simulink model "hydraulic_nonlin_stud"  (R2025b)
settings: Solver=ode4  StartTime=0.0  StopTime=30  FixedStep=0.001  RelTol=1e-3
values from neighbouring files (symbols this model uses):
  A = real(A)    [untitled.m]
  B = real(B)    [untitled.m]
  C = [1 0 0 0]    [untitled.m]
  D = 0    [untitled.m]
  k = real(k)    [untitled.m]
  N = real(N)    [untitled.m]
libraries: simulink x1
settings Model: Creator=Zsofi  LastModifiedBy=User
settings SolverCC: AlgebraicLoopSolver=TrustRegion
settings DataIOCC: SaveFormat=StructureWithTime  ReturnWorkspaceOutputs=off
settings OptimizationCC: LifeSpan=inf
settings DebuggingCC: FcnCallInpInsideContextMsg=warning  UnconnectedInputMsg=warning  UnconnectedOutputMsg=warning  UnconnectedLineMsg=warning  SFExecutionAtInitializationDiag=none  ArithmeticOperatorsInVariantConditions=warning
settings HardwareCC: ProdBitPerSizeT=32.0  ProdBitPerPtrDiffT=32.0  ProdWordSize=32.0  ProdHWDeviceType=Specified
settings ModelReferenceCC: EnableRefExpFcnMdlSchedulingChecks=on
settings SFSimCC: SimUseLocalCustomCode=off  CustomCodeUndefinedFunction=UseInterfaceOnly
settings RTWCC: RTWUseLocalCustomCode=off  GPUComputeCapability=3.5
settings CodeAppCC: StateflowObjectComments=on

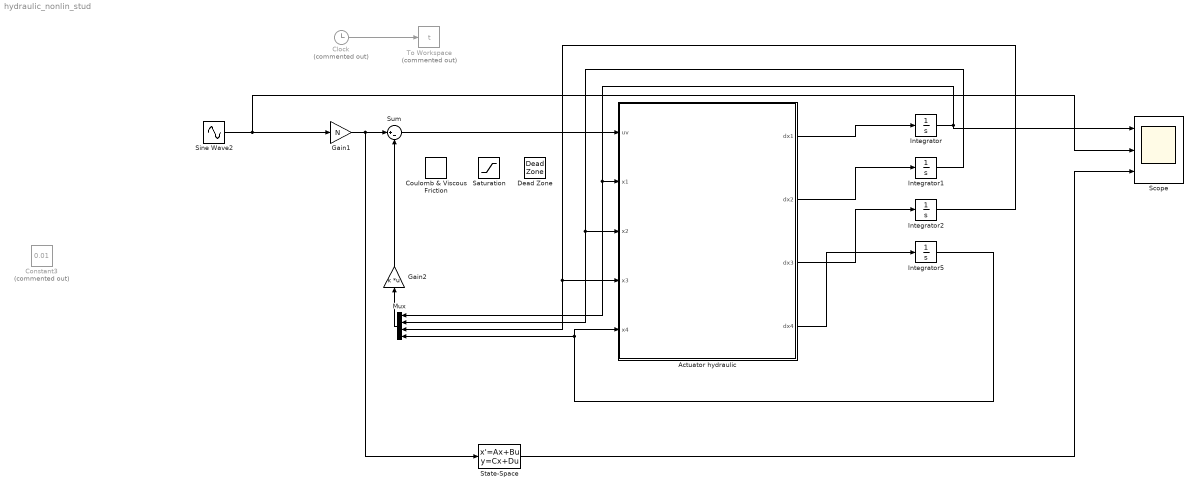
== system hydraulic_nonlin_stud ==
  Actuator hydraulic : MATLAB Function  TreatAsAtomicUnit=on
  Clock : Clock  Commented=on
  Constant3 : Constant  Commented=on  Value=0.01
  Coulomb & Viscous Friction : simulink/Discontinuities/Coulomb & Viscous Friction  offset=[0.005]  gain=1
  Dead Zone : DeadZone  LowerValue=-0.005  UpperValue=0.005
  Gain1 : Gain  Gain=N
  Gain2 : Gain  Gain=k  Multiplication=Matrix(K*u)
  Integrator{,1..2,5} (4 alike) : Integrator
  Mux : Mux
  Saturation : Saturate  UpperLimit=0.1  LowerLimit=-0.1
  Scope : Scope  NumInputPorts=3
      settings: ActiveDisplayYMinimum=-0.024999999679969208  ActiveDisplayYMaximum=0.024999999961916909
  Sine Wave2 : Sin  Amplitude=0.02  Frequency=10  SampleTime=0
  State-Space : StateSpace  A=A-B*k  B=B  C=C  D=D  InitialCondition=0
  Sum : Sum  Inputs=|+-
  To Workspace : ToWorkspace  Commented=on  VariableName=t  SampleTime=-1
  wires:
  Clock/1 -> To Workspace/1
  Actuator hydraulic/1(dx1) -> Integrator/1
  Integrator/1 -> Scope/1, Mux/1, Actuator hydraulic/2(x1)
  Integrator1/1 -> Mux/2, Actuator hydraulic/3(x2)
  Actuator hydraulic/2(dx2) -> Integrator1/1
  Integrator2/1 -> Actuator hydraulic/4(x3), Mux/3
  Actuator hydraulic/3(dx3) -> Integrator2/1
  Sine Wave2/1 -> Scope/2, Gain1/1
  Actuator hydraulic/4(dx4) -> Integrator5/1
  Integrator5/1 -> Mux/4, Actuator hydraulic/5(x4)
  Gain1/1 -> State-Space/1, Sum/1
  Mux/1 -> Gain2/1
  Gain2/1 -> Sum/2
  Sum/1 -> Actuator hydraulic/1(uv)
  State-Space/1 -> Scope/3

== matlab function hydraulic_nonlin_stud/Actuator hydraulic ==
  data: uv input; dx1 output; dx2 output; dx3 output; dx4 output; x1 input; x2 input; x3 input; x4 input
function [dx1, dx2, dx3, dx4] = fcn(uv, x1, x2, x3, x4)
M = 10.8;    
Bv = 13.1;   
L0 = 0.1635; 
b = 1.04;    
Kg = 1.035;  
gamma = 1.4; 
R = 287;     
T = 293;     
RT = R*T;
Patm = 101325; 
Ps = 600000;   
P0 = 300000;   
cv = 0.024;    

%iesiri
dx1 = 0; dx2 = 0; dx3 = 0; dx4 = 0;

% limite sigure pentru comanda de intrare directa
if uv > 10
    uv_safe = 10;     % limitare +10V
elseif uv < -10
    uv_safe = -10;    % limitare -10V
else
    uv_safe = uv;     % comanda in interval sigur
end

if x1 > 0.05
    x1_limited = 0.05;   % +5 cm
elseif x1 < -0.05
    x1_limited = -0.05;  % -5 cm
else
    x1_limited = x1;     
end

La = L0 + x1_limited; 
Lb = L0 - x1_limited;

Va = max(1e-4, (La * (b^2 - (La^2))) / Kg);
Vb = max(1e-4, (Lb * (b^2 - (Lb^2))) / Kg); 

dVadx = (b^2 - 3*(La^2)) / Kg;
dVbdx = -(b^2 - 3*(Lb^2)) / Kg; 

% debite si presiuni
% se imparte cu 1e5 pt a se potrivi cu unitatile
qmA = cv * uv_safe * sqrt(max(0, Ps - P0)/1e5);
qmB = -cv * uv_safe * sqrt(max(0, P0 - Patm)/1e5);

% dinamica presiunilor individuale
dPa = (gamma * RT * qmA) / Va - (gamma * P0 / Va) * dVadx * x2;
dPb = (gamma * RT * qmB) / Vb - (gamma * P0 / Vb) * dVbdx * x2; 
dPd = dPa - dPb;

% dinamica mecanica
F_pneuma = x4 * dVadx;
dacc_mecanic = (1/M) * (F_pneuma - Bv * x3);

% atribuire finala a derivatelor
dx1 = x2;
dx2 = x3;
dx3 = dacc_mecanic;
dx4 = dPd;
